simulink model "flightController"  (R2021a)
settings: Solver=ode3  StartTime=0  StopTime=10  FixedStep=Ts  RelTol=1e-3  EnableMultiTasking=on
undefined symbols (not defined in the file): Controller, ControlvsRed, D_ROLL, delays, DiscIntNeverNeededParam, g, I_ROLL, norm_act, Normalization, P_Pitch, P_ROLL, P_Roll, P_Yaw, P_z, PR_Start, save_time, sts_cnames, time_DisYaw, time_stepsX, time_stepsY, time_stepsZ, Ts, Vehicle, x0, x0_f
libraries: deeplib x5
(part 1 of 4)
settings Model: Creator=The MathWorks, Inc.  LastModifiedBy=Eduardo
settings SolverCC: AlgebraicLoopSolver=TrustRegion  MinimalZcImpactIntegration=on
settings DataIOCC: LimitDataPoints=on  SaveFormat=Array  ReturnWorkspaceOutputs=off
settings OptimizationCC: BlockReduction=off  DefaultParameterBehavior=Inlined  BufferReuse=off  PassReuseOutputArgsThreshold=0
settings DebuggingCC: AlgebraicLoopMsg=none  ParameterPrecisionLossMsg=none  ParameterTunabilityLossMsg=error  UnconnectedInputMsg=none  UnconnectedOutputMsg=none  UnconnectedLineMsg=none  BusObjectLabelMismatch=error  SFUnexpectedBacktrackingDiag=warning  SFNoUnconditionalDefaultTransitionDiag=warning  SFExecutionAtInitializationDiag=none  SFMachineParentedDataDiag=warning  ArithmeticOperatorsInVariantConditions=warning
settings HardwareCC: ProdBitPerPointer=32  ProdBitPerSizeT=32  ProdBitPerPtrDiffT=32  ProdLargestAtomicInteger=Long  ProdWordSize=32  ProdHWDeviceType=ARM Compatible->ARM 9
settings ModelReferenceCC: ModelReferenceNumInstancesAllowed=Single  PropagateSignalLabelsOutOfModel=off
settings SFSimCC: SimUseLocalCustomCode=off  CustomCodeUndefinedFunction=UseInterfaceOnly
settings RTWCC: Description=Generic Real-Time Target  GenerateReport=on  RTWUseLocalCustomCode=off  LaunchReport=on
settings CodeAppCC: ForceParamTrailComments=on  MaxIdLength=63  OperatorAnnotations=on  StateflowObjectComments=on  MATLABSourceComments=on
settings GRTTargetCC: TargetLangStandard=C89/C90 (ANSI)
settings ConfigComp: CovMetricSettings=dw  CovSaveCumulativeToWorkspaceVar=on  CovSaveSingleToWorkspaceVar=on  CovExternalEMLEnable=off  CovSFcnEnable=off

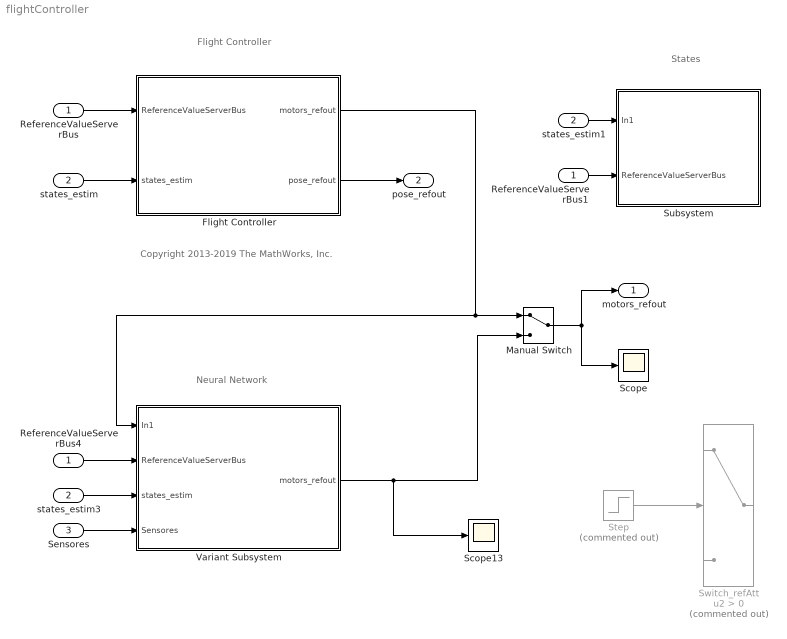
== system flightController ==
  note: States
  note: Copyright 2013-2019 The MathWorks, Inc.
  note: Neural Network
  note: Flight Controller
  ReferenceValueServerBus : Inport  OutDataTypeStr=Bus: CommandBus  BusOutputAsStruct=on
  states_estim : Inport  Port=2  OutDataTypeStr=Bus: statesEstim_t  BusOutputAsStruct=on
  Sensores : Inport  Port=3  OutDataTypeStr=Bus: sensordata_t
  Flight Controller : Subsystem
  Manual Switch : ManualSwitch
  ReferenceValueServerBus1 : InportShadow  OutDataTypeStr=Bus: CommandBus  BusOutputAsStruct=on
  ReferenceValueServerBus4 : InportShadow  OutDataTypeStr=Bus: CommandBus  BusOutputAsStruct=on
  Scope : Scope
  Scope13 : Scope
  Step : Step  Commented=on  Time=0  After=ControlvsRed
  Subsystem : Subsystem
  Switch_refAtt : Switch  Commented=on  Criteria=u2 > Threshold
  Variant Subsystem : Subsystem  Variant=on
  states_estim1 : InportShadow  Port=2  OutDataTypeStr=Bus: statesEstim_t  BusOutputAsStruct=on
  states_estim3 : InportShadow  Port=2  OutDataTypeStr=Bus: statesEstim_t  BusOutputAsStruct=on
  motors_refout : Outport  VectorParamsAs1DForOutWhenUnconnected=off
  pose_refout : Outport  Port=2  VectorParamsAs1DForOutWhenUnconnected=off
  wires:
  ReferenceValueServerBus/1 -> Flight Controller/1(ReferenceValueServerBus)
  states_estim/1 -> Flight Controller/2(states_estim)
  Flight Controller/2(pose_refout) -> pose_refout/1
  Manual Switch/1 -> motors_refout/1, Scope/1
  Flight Controller/1(motors_refout) -> Variant Subsystem/1(In1), Manual Switch/1
  Step/1 -> Switch_refAtt/2
  Variant Subsystem/1(motors_refout) -> Manual Switch/2, Scope13/1
  ReferenceValueServerBus4/1 -> Variant Subsystem/2(ReferenceValueServerBus)
  states_estim3/1 -> Variant Subsystem/3(states_estim)
  Sensores/1 -> Variant Subsystem/4(Sensores)
  ReferenceValueServerBus1/1 -> Subsystem/2(ReferenceValueServerBus)
  states_estim1/1 -> Subsystem/1(In1)

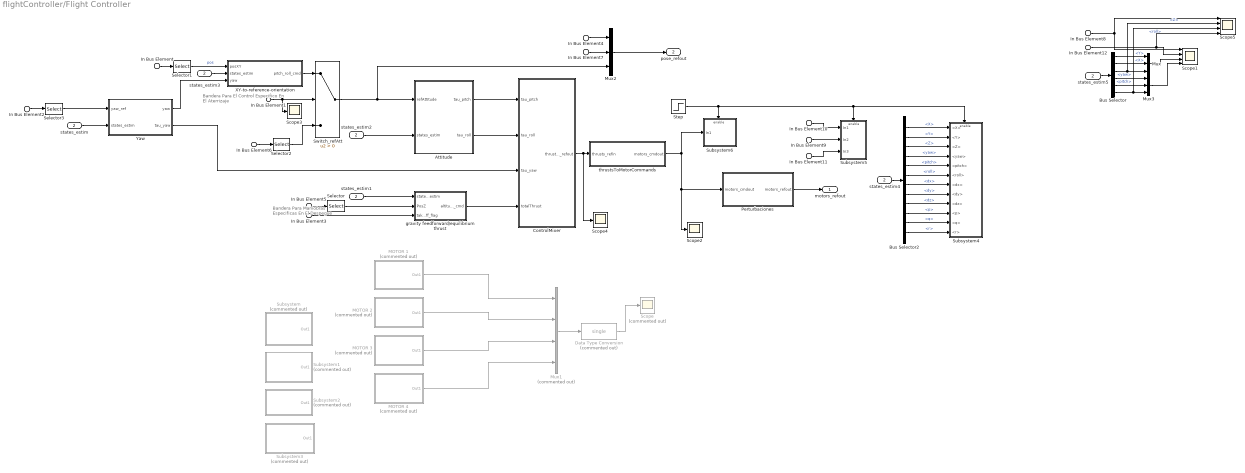
== system flightController/Flight Controller ==
  note: Bandera Para El Control
      | Especifico En El Aterrizaje
  note: Bandera Para
      | Maniobras
      | Especificas
      | En El Despegue
  In Bus Element1 : Inport  PortName=ReferenceValueServerBus  Element=controlModePosVSOrient
  In Bus Element11 : Inport  PortName=ReferenceValueServerBus  Element=controlModePosVSOrient
  In Bus Element{,4..5,8..9} (5 alike) : Inport  PortName=ReferenceValueServerBus  Element=pos_ref
  In Bus Element{2,6..7,10,12} (5 alike) : Inport  PortName=ReferenceValueServerBus  Element=orient_ref
  In Bus Element3 : Inport  PortName=ReferenceValueServerBus  Element=takeoff_flag
  states_estim : Inport  Port=2
  Attitude : Subsystem
  Bus Selector : BusSelector  OutputSignals=Y,X,Z,yaw,pitch,roll
  Bus Selector2 : BusSelector  OutputSignals=X,Y,Z,yaw,pitch,roll,dx,dy,dz,p,q,r
  ControlMixer : Subsystem
  Data Type Conversion : DataTypeConversion  Commented=on  OutDataTypeStr=single
  "MOTOR 1 " : Subsystem  Commented=on  Variant=on  VariantControlMode=label  LabelModeActiveChoice=Choice
  MOTOR 2 : Subsystem  Commented=on  Variant=on  VariantControlMode=label  LabelModeActiveChoice=Choice
  "MOTOR 3 " : Subsystem  Commented=on  Variant=on  VariantControlMode=label  LabelModeActiveChoice=Choice
  "MOTOR 4 " : Subsystem  Commented=on  Variant=on  VariantControlMode=label  LabelModeActiveChoice=Choice
  Mux : Mux  Inputs=3
  Mux1 : Mux  Commented=on
  Mux2 : Mux  Inputs=3
  Mux3 : Mux  Inputs=3
  Perturbaciones : Subsystem
  Scope : Scope  Commented=on
  Scope1 : Scope  NumInputPorts=4
  Scope2 : Scope
  Scope3 : Scope
  Scope4 : Scope
  Scope5 : Scope  NumInputPorts=4
  Selector : Selector  InputPortWidth=3  IndexOptions=Index vector (dialog)  Indices=3  OutputSizes=1
  Selector1 : Selector  InputPortWidth=3  IndexOptions=Index vector (dialog)  Indices=[1 2]  OutputSizes=1
  Selector2 : Selector  InputPortWidth=3  IndexOptions=Index vector (dialog)  Indices=[2 3]  OutputSizes=1
  Selector3 : Selector  InputPortWidth=3  IndexOptions=Index vector (dialog)  Indices=1  OutputSizes=1
  Step : Step  Time=save_time
  Subsystem : Subsystem  Commented=on
  Subsystem1 : Subsystem  Commented=on
  Subsystem2 : Subsystem  Commented=on
  Subsystem3 : Subsystem  Commented=on
  Subsystem4 : Subsystem
  Subsystem5 : Subsystem
  Subsystem6 : Subsystem
  Switch_refAtt : Switch  Criteria=u2 > Threshold
  XY-to-reference-orientation : Subsystem
  Yaw : Subsystem
  gravity feedforward/equilibrium thrust : Subsystem
  states_estim{1..5} (5 alike) : InportShadow  Port=2
  thrustsToMotorCommands : Subsystem
  motors_refout : Outport  VectorParamsAs1DForOutWhenUnconnected=off
  pose_refout : Outport  Port=2  VectorParamsAs1DForOutWhenUnconnected=off
  wires:
  In Bus Element1/1 -> Scope3/1, Switch_refAtt/2
  XY-to-reference-orientation/1(pitch_roll_cmd) -> Switch_refAtt/1
  In Bus Element2/1 -> Selector3/1
  In Bus Element/1 -> Selector1/1
  Selector3/1 -> Yaw/1(yaw_ref)
  Selector1/1 -> XY-to-reference-orientation/1(posXY)  "pos"
  ControlMixer/1(thrusts_refout) -> thrustsToMotorCommands/1(thrusts_refin), Scope4/1
  states_estim/1 -> Yaw/2(states_estim)
  Switch_refAtt/1 -> Attitude/1(refAttitude), Mux2/3
  Yaw/1(yaw) -> XY-to-reference-orientation/3(yaw)
  gravity feedforward/equilibrium thrust/1(altitude_cmd) -> ControlMixer/4(totalThrust)
  Attitude/1(tau_pitch) -> ControlMixer/1(tau_pitch)
  Attitude/2(tau_roll) -> ControlMixer/2(tau_roll)
  Yaw/2(tau_yaw) -> ControlMixer/3(tau_yaw)
  states_estim1/1 -> gravity feedforward/equilibrium thrust/1(states_estim)
  states_estim2/1 -> Attitude/2(states_estim)
  states_estim3/1 -> XY-to-reference-orientation/2(states_estim)
  In Bus Element4/1 -> Mux2/1
  Selector/1 -> gravity feedforward/equilibrium thrust/2(PosZ)
  In Bus Element5/1 -> Selector/1
  In Bus Element6/1 -> Selector2/1
  Selector2/1 -> Switch_refAtt/3
  In Bus Element7/1 -> Mux2/2
  Mux1/1 -> Data Type Conversion/1
  "MOTOR 1 "/1(Out1) -> Mux1/1
  MOTOR 2/1(Out1) -> Mux1/2
  "MOTOR 3 "/1(Out1) -> Mux1/3
  "MOTOR 4 "/1(Out1) -> Mux1/4
  Mux2/1 -> pose_refout/1
  Data Type Conversion/1 -> Scope/1
  states_estim4/1 -> Bus Selector2/1
  In Bus Element8/1 -> Scope5/1, Scope1/1
  states_estim5/1 -> Bus Selector/1
  Bus Selector/1 -> Mux/1  "<Y>"
  Bus Selector/3 -> Scope5/2, Mux/3  "<Z>"
  Bus Selector/4 -> Mux3/1  "<yaw>"
  Bus Selector/5 -> Mux3/2  "<pitch>"
  Bus Selector/6 -> Scope5/3, Mux3/3  "<roll>"
  In Bus Element3/1 -> gravity feedforward/equilibrium thrust/3(takeoff_flag)
  Bus Selector2/1 -> Subsystem4/1(<X>)  "<X>"
  Bus Selector2/2 -> Subsystem4/2(<Y>)  "<Y>"
  Bus Selector2/3 -> Subsystem4/3(<Z>)  "<Z>"
  Bus Selector2/4 -> Subsystem4/4(<yaw>)  "<yaw>"
  Bus Selector2/5 -> Subsystem4/5(<pitch>)  "<pitch>"
  Bus Selector2/6 -> Subsystem4/6(<roll>)  "<roll>"
  Bus Selector2/7 -> Subsystem4/7(<dx>)  "<dx>"
  Bus Selector2/8 -> Subsystem4/8(<dy>)  "<dy>"
  Bus Selector2/9 -> Subsystem4/9(<dz>)  "<dz>"
  Bus Selector2/10 -> Subsystem4/10(<p>)  "<p>"
  Bus Selector2/11 -> Subsystem4/11(<q>)  "<q>"
  Bus Selector2/12 -> Subsystem4/12(<r>)  "<r>"
  Step/1 -> Subsystem6/Enable, Subsystem5/Enable, Subsystem4/Enable
  In Bus Element10/1 -> Subsystem5/1(In1)
  In Bus Element9/1 -> Subsystem5/2(In2)
  In Bus Element11/1 -> Subsystem5/3(In3)
  In Bus Element12/1 -> Scope5/4, Scope1/2
  thrustsToMotorCommands/1(motors_cmdout) -> Perturbaciones/1(motors_cmdout), Scope2/1, Subsystem6/1(In1)
  Bus Selector/2 -> Mux/2  "<X>"
  Mux/1 -> Scope1/3
  Mux3/1 -> Scope1/4
  Perturbaciones/1(motors_refout) -> motors_refout/1

== system flightController/Subsystem ==
  note: Yaw
  note: X
  note: Y
  note: Z
  note: Pitch
  note: Roll
  In1 : Inport
  In Bus Element2 : Inport  Port=2  PortName=ReferenceValueServerBus  Element=orient_ref
  In Bus Element5 : Inport  Port=2  PortName=ReferenceValueServerBus  Element=orient_ref
  In Bus Element6 : Inport  Port=2  PortName=ReferenceValueServerBus  Element=orient_ref
  In Bus Element1 : Inport  Port=2  PortName=ReferenceValueServerBus  Element=pos_ref
  In Bus Element3 : Inport  Port=2  PortName=ReferenceValueServerBus  Element=pos_ref
  In Bus Element4 : Inport  Port=2  PortName=ReferenceValueServerBus  Element=pos_ref
  Bus Selector2 : BusSelector  OutputSignals=X,Y,Z,yaw,pitch,roll
  Mux{,1..5} (6 alike) : Mux  Inputs=2
  Scope1 : Scope  NumInputPorts=6
  Selector1 : Selector  InputPortWidth=3  IndexOptions=Index vector (dialog)  Indices=1  OutputSizes=1
  Selector2 : Selector  InputPortWidth=3  IndexOptions=Index vector (dialog)  Indices=2  OutputSizes=1
  Selector3 : Selector  InputPortWidth=3  IndexOptions=Index vector (dialog)  Indices=1  OutputSizes=1
  Selector4 : Selector  InputPortWidth=3  IndexOptions=Index vector (dialog)  Indices=3  OutputSizes=1
  Selector5 : Selector  InputPortWidth=3  IndexOptions=Index vector (dialog)  Indices=2  OutputSizes=1
  Selector6 : Selector  InputPortWidth=3  IndexOptions=Index vector (dialog)  Indices=3  OutputSizes=1
  wires:
  In Bus Element2/1 -> Selector3/1
  In1/1 -> Bus Selector2/1
  Bus Selector2/1 -> Mux/1  "<X>"
  Bus Selector2/2 -> Mux1/1  "<Y>"
  Bus Selector2/3 -> Mux2/1  "<Z>"
  Bus Selector2/4 -> Mux3/1  "<yaw>"
  Bus Selector2/5 -> Mux4/1  "<pitch>"
  Bus Selector2/6 -> Mux5/1  "<roll>"
  In Bus Element1/1 -> Selector1/1
  In Bus Element3/1 -> Selector2/1
  In Bus Element4/1 -> Selector4/1
  In Bus Element5/1 -> Selector5/1
  In Bus Element6/1 -> Selector6/1
  Selector1/1 -> Mux/2  "X_ref"
  Selector2/1 -> Mux1/2  "Y_ref"
  Selector4/1 -> Mux2/2  "Z_ref"
  Selector3/1 -> Mux3/2  "Yaw_ref"
  Selector5/1 -> Mux4/2  "Pitch_ref"
  Selector6/1 -> Mux5/2  "Roll_ref"
  Mux/1 -> Scope1/1
  Mux2/1 -> Scope1/3
  Mux5/1 -> Scope1/6
  Mux4/1 -> Scope1/5
  Mux3/1 -> Scope1/4
  Mux1/1 -> Scope1/2

== system flightController/Variant Subsystem ==
  note: 1) Add Subsystem or Model blocks as valid variant choices.
      | 2) You cannot connect blocks at this level. At simulation, connectivity is automatically
      | determined, based on the active variant and port name matching.
  In1 : Inport
  ReferenceValueServerBus : Inport  Port=2
  states_estim : Inport  Port=3
  Sensores : Inport  Port=4
  ANN : Subsystem  VariantControl=ANN
  ANN_Feedback : Subsystem  VariantControl=ANN_Feedback
  LSTM : Subsystem  VariantControl=LSTM
  motors_refout : Outport

== system flightController/Flight Controller/Attitude ==
  note: [0.002;0.01119]
  note: 0.001616
  note: OC [P]
  note: OPSO [P]
  note: [0.013;0.06656]
  note: 0.005
  note: [0.013;0.01]
  note: [0.002; 0.0028]
  note: 0.001
  note: OC [I]
  note: ATTITUDE
  note: 0.01
  note: OPSO [I]
  note: OC [D]
  note: OPSO [D]
  refAttitude : Inport
  states_estim : Inport  Port=2
  Add : Sum  Inputs=+-
  Bus Selector3 : BusSelector  OutputSignals=pitch,roll
  Bus Selector4 : BusSelector  OutputSignals=q,p
  D_pr : Gain  Gain=[0.002; D_ROLL]
  Delay : Delay  DelayLength=1  InitialCondition=0
  Demux : Demux  Outputs=2
  Discrete-Time Integrator : DiscreteIntegrator  SampleTime=Ts  LimitOutput=on  UpperSaturationLimit=2  LowerSaturationLimit=-2  ICPrevOutput=DiscIntNeverNeededParam  ICPrevScaledInput=DiscIntNeverNeededParam
  I_pr : Gain  Gain=I_ROLL
  Mux : Mux  Inputs=2
  Mux1 : Mux  Inputs=2
  P_pr : Gain  Gain=[0.013;P_ROLL]
  Scope : Scope
  Scope{1..5} (5 alike) : Scope  NumInputPorts=2
  Sum16 : Sum  Inputs=++-  AccumDataTypeStr=single  OutDataTypeStr=single  SaturateOnIntegerOverflow=on
  Sum19 : Sum  Inputs=+-|
  antiWU_Gain : Gain  Gain=0.001
  tau_pitch : Outport  VectorParamsAs1DForOutWhenUnconnected=off
  tau_roll : Outport  Port=2  VectorParamsAs1DForOutWhenUnconnected=off
  wires:
  Sum16/1 -> Demux/1  "P_pr"
  antiWU_Gain/1 -> Add/2
  Add/1 -> Discrete-Time Integrator/1
  Bus Selector3/1 -> Mux/1  "<pitch>"
  Bus Selector4/1 -> Mux1/1  "<q>"
  P_pr/1 -> Scope3/2, Sum16/1
  I_pr/1 -> Sum16/2, Scope/1
  Sum19/1 -> Add/1, Scope2/2, P_pr/1  "pitch/roll error"
  Discrete-Time Integrator/1 -> Delay/1, I_pr/1
  Delay/1 -> antiWU_Gain/1
  Demux/1 -> tau_pitch/1  "tau_pitch"
  Demux/2 -> tau_roll/1
  D_pr/1 -> Scope5/1, Sum16/3
  states_estim/1 -> Bus Selector3/1, Bus Selector4/1
  refAttitude/1 -> Sum19/1
  Mux/1 -> Sum19/2
  Bus Selector3/2 -> Scope1/1, Mux/2  "<roll>"
  Mux1/1 -> Scope4/1, D_pr/1
  Bus Selector4/2 -> Scope1/2, Mux1/2  "<p>"

== system flightController/Flight Controller/ControlMixer ==
  tau_pitch : Inport
  tau_roll : Inport  Port=2
  tau_yaw : Inport  Port=3
  totalThrust : Inport  Port=4
  Mux2 : Mux
  Product : Product  Multiplication=Matrix(*)  RndMeth=Zero
  TorqueTotalThrustToThrustPerMotor : Constant  Value=Controller.Q2Ts  OutDataTypeStr=single
  thrusts_refout : Outport  VectorParamsAs1DForOutWhenUnconnected=off
  wires:
  Product/1 -> thrusts_refout/1
  tau_roll/1 -> Mux2/4
  tau_pitch/1 -> Mux2/3
  tau_yaw/1 -> Mux2/2
  totalThrust/1 -> Mux2/1
  TorqueTotalThrustToThrustPerMotor/1 -> Product/1
  Mux2/1 -> Product/2

== system flightController/Flight Controller/MOTOR 1  ==
  note: 1) Add Subsystem or Model blocks as valid variant choices.
      | 2) You cannot connect blocks at this level. At simulation, connectivity is automatically
      | determined, based on the active variant and port name matching.
  "PITCH " : Subsystem  VariantControl=Choice_3
  "ROLL " : Subsystem  VariantControl=Choice
  SUBIR : Subsystem  VariantControl=Choice_1
  YAW : Subsystem  VariantControl=Choice_2
  Out1 : Outport

== system flightController/Flight Controller/MOTOR 2 ==
  note: 1) Add Subsystem or Model blocks as valid variant choices.
      | 2) You cannot connect blocks at this level. At simulation, connectivity is automatically
      | determined, based on the active variant and port name matching.
  "PITCH " : Subsystem  VariantControl=Choice_3
  ROLL : Subsystem  VariantControl=Choice
  SUBIR : Subsystem  VariantControl=Choice_1
  YAW : Subsystem  VariantControl=Choice_2
  Out1 : Outport

== system flightController/Flight Controller/MOTOR 3  ==
  note: 1) Add Subsystem or Model blocks as valid variant choices.
      | 2) You cannot connect blocks at this level. At simulation, connectivity is automatically
      | determined, based on the active variant and port name matching.
  "PITCH " : Subsystem  VariantControl=Choice_3
  "ROLL " : Subsystem  VariantControl=Choice
  SUBIR : Subsystem  VariantControl=Choice_1
  YAW : Subsystem  VariantControl=Choice_2
  Out1 : Outport

== system flightController/Flight Controller/MOTOR 4  ==
  note: 1) Add Subsystem or Model blocks as valid variant choices.
      | 2) You cannot connect blocks at this level. At simulation, connectivity is automatically
      | determined, based on the active variant and port name matching.
  "PITCH " : Subsystem  VariantControl=Choice_3
  "ROLL " : Subsystem  VariantControl=Choice
  SUBIR : Subsystem  VariantControl=Choice_1
  YAW : Subsystem  VariantControl=Choice_2
  Out1 : Outport

== system flightController/Flight Controller/Perturbaciones ==
  motors_cmdout : Inport
  Data Type Conversion : DataTypeConversion  OutDataTypeStr=single
  Demux : Demux
  Mux1 : Mux
  Perturbaciones en Pitch : Subsystem
  Perturbaciones en Roll : Subsystem
  Perturbaciones en Yaw : Subsystem
  Perturbaciones en Z : Subsystem
  Scope6 : Scope  NumInputPorts=4
  Sum : Sum  Inputs=|++++
  Sum1 : Sum  Inputs=|++-+
  Sum2 : Sum  Inputs=|++
  Sum3 : Sum  Inputs=|++-+
  motors_refout : Outport
  wires:
  Perturbaciones en Z/1(Out1) -> Sum1/3, Sum/4, Sum2/2, Sum3/3
  Mux1/1 -> Data Type Conversion/1
  Demux/4 -> Sum3/1
  Demux/1 -> Sum/1
  Perturbaciones en Roll/1(Out1) -> Sum/3, Sum1/2, Scope6/4
  Sum2/1 -> Mux1/3
  Sum3/1 -> Mux1/4
  Perturbaciones en Pitch/1(Out1) -> Scope6/2, Sum3/2, Sum/2, Scope6/1
  Sum1/1 -> Mux1/2
  Demux/2 -> Sum1/1
  Demux/3 -> Sum2/1
  Sum/1 -> Mux1/1
  motors_cmdout/1 -> Demux/1
  Data Type Conversion/1 -> motors_refout/1
  Perturbaciones en Yaw/1(Out1) -> Scope6/3, Sum3/4, Sum1/4

== system flightController/Flight Controller/Subsystem ==
  note: SI
  Pulse Generator : DiscretePulseGenerator  Commented=on  PulseType=Time based  Amplitude=50  Period=1.5  PulseWidth=50
  Pulse Generator1 : DiscretePulseGenerator  Commented=on  PulseType=Time based  Amplitude=30  Period=1.5  PulseWidth=50
  Step : Step  Commented=on  Time=0.001  Before=30  After=350
  Step1 : Step  Commented=on  Time=0.001  Before=30  After=350
  Step10 : Step  Commented=on  Time=0.001  Before=30  After=380
  Step11 : Step  Commented=on  Time=1.5  Before=1  After=0
  Step2 : Step  Commented=on  Time=0.001  Before=30  After=420
  Step3 : Step  Commented=on  Time=1.5  Before=1  After=0
  Step4 : Step  Commented=on  Time=0.001  Before=-30  After=237
  Step5 : Step  Commented=on  Time=3  Before=1  After=0
  Step6 : Step  Time=0.001  Before=30  After=350
  Step7 : Step  Time=0.001  Before=30  After=380
  Step8 : Step  Time=1.5  Before=1  After=0
  Step9 : Step  Commented=on  Time=0.001  Before=30  After=350
  Sum : Sum  Commented=on  Inputs=|+-
  Sum1 : Sum  Commented=on  Inputs=|+-
  Switch : Switch  Commented=on  Criteria=u2 > Threshold
  Switch1 : Switch  Commented=on  Criteria=u2 > Threshold
  Switch2 : Switch  Criteria=u2 > Threshold
  Switch3 : Switch  Commented=on  Criteria=u2 > Threshold
  Out1 : Outport
  wires:
  Step/1 -> Switch/1
  Step5/1 -> Switch/2
  Pulse Generator/1 -> Sum/2
  Step2/1 -> Sum/1
  Sum/1 -> Switch/3
  Step1/1 -> Switch1/1
  Step3/1 -> Switch1/2
  Step4/1 -> Sum1/1
  Sum1/1 -> Switch1/3
  Pulse Generator1/1 -> Sum1/2
  Step6/1 -> Switch2/1
  Step8/1 -> Switch2/2
  Step7/1 -> Switch2/3
  Step11/1 -> Switch3/2
  Step10/1 -> Switch3/3
  Step9/1 -> Switch3/1
  Switch2/1 -> Out1/1

== system flightController/Flight Controller/Subsystem1 ==
  note: SI
  Pulse Generator : DiscretePulseGenerator  Commented=on  PulseType=Time based  Amplitude=50  Period=1.5  PulseWidth=50
  Pulse Generator1 : DiscretePulseGenerator  Commented=on  PulseType=Time based  Amplitude=30  Period=1.5  PulseWidth=50
  Step1 : Step  Commented=on  Time=0.001  Before=-30  After=-280
  Step10 : Step  Commented=on  Time=0.001  Before=-30  After=-310
  Step{2,4,8,11} (4 alike) : Step  Commented=on  Time=0.001  Before=-30  After=-350
  Step12 : Step  Commented=on  Time=1.5
  Step3 : Step  Commented=on  Time=3
  Step5 : Step  Commented=on  Time=1.5
  Step6 : Step  Commented=on  Time=0.001  Before=-30  After=-380
  Step7 : Step  Commented=on  Time=0.001  Before=-30  After=-237
  Step9 : Step  Commented=on  Time=1.5
  Sum : Sum  Commented=on  Inputs=|++
  Sum1 : Sum  Commented=on  Inputs=|++
  Switch{,1..3} (4 alike) : Switch  Commented=on  Criteria=u2 > Threshold
  Out1 : Outport
  wires:
  Step5/1 -> Switch/2
  Step4/1 -> Switch/3
  Sum1/1 -> Switch/1
  Step3/1 -> Switch1/2
  Step2/1 -> Switch1/3
  Pulse Generator/1 -> Sum/1
  Step1/1 -> Sum/2
  Sum/1 -> Switch1/1
  Pulse Generator1/1 -> Sum1/2
  Step7/1 -> Sum1/1
  Step8/1 -> Switch2/3
  Step6/1 -> Switch2/1
  Step9/1 -> Switch2/2
  Step12/1 -> Switch3/2
  Step11/1 -> Switch3/3
  Step10/1 -> Switch3/1
  Switch1/1 -> Out1/1

== system flightController/Flight Controller/Subsystem2 ==
  note: SI
  Pulse Generator : DiscretePulseGenerator  PulseType=Time based  Amplitude=50  Period=1.5  PulseWidth=50
  Pulse Generator1 : DiscretePulseGenerator  Commented=on  PulseType=Time based  Amplitude=30  Period=1.5  PulseWidth=50
  Step : Step  Commented=on  Time=0.001  Before=30  After=350
  Step1 : Step  Time=0.001  Before=30  After=350
  Step10 : Step  Commented=on  Time=0.001  Before=30  After=310
  Step11 : Step  Commented=on  Time=1.5  Before=1  After=0
  Step2 : Step  Time=0.001  Before=30  After=420
  Step3 : Step  Time=3  Before=1  After=0
  Step4 : Step  Commented=on  Time=0.001  Before=-30  After=237
  Step5 : Step  Commented=on  Time=1.5  Before=1  After=0
  Step6 : Step  Commented=on  Time=0.001  Before=30  After=350
  Step7 : Step  Commented=on  Time=0.001  Before=30  After=310
  Step8 : Step  Commented=on  Time=1.5  Before=1  After=0
  Step9 : Step  Commented=on  Time=0.001  Before=30  After=350
  Sum : Sum  Inputs=|+-
  Sum1 : Sum  Commented=on  Inputs=|+-
  Switch : Switch  Commented=on  Criteria=u2 > Threshold
  Switch1 : Switch  Criteria=u2 > Threshold
  Switch2 : Switch  Commented=on  Criteria=u2 > Threshold
  Switch3 : Switch  Commented=on  Criteria=u2 > Threshold
  Out1 : Outport
  wires:
  Step5/1 -> Switch/2
  Step/1 -> Switch/1
  Step1/1 -> Switch1/1
  Step3/1 -> Switch1/2
  Step2/1 -> Sum/1
  Sum/1 -> Switch1/3
  Pulse Generator/1 -> Sum/2
  Pulse Generator1/1 -> Sum1/2
  Step4/1 -> Sum1/1
  Sum1/1 -> Switch/3
  Step8/1 -> Switch2/2
  Step6/1 -> Switch2/1
  Step7/1 -> Switch2/3
  Step9/1 -> Switch3/1
  Step11/1 -> Switch3/2
  Step10/1 -> Switch3/3
  Switch1/1 -> Out1/1

== system flightController/Flight Controller/Subsystem3 ==
  note: SI
  Pulse Generator : DiscretePulseGenerator  PulseType=Time based  Amplitude=50  Period=1.5  PulseWidth=50
  Pulse Generator1 : DiscretePulseGenerator  Commented=on  PulseType=Time based  Amplitude=30  Period=1.5  PulseWidth=50
  Step1 : Step  Time=0.001  Before=-30  After=-280
  Step10 : Step  Commented=on  Time=0.001  Before=-30  After=-380
  Step11 : Step  Commented=on  Time=0.001  Before=-30  After=-350
  Step12 : Step  Commented=on  Time=1.5
  Step2 : Step  Time=0.001  Before=-30  After=-350
  Step3 : Step  Time=3
  Step4 : Step  Commented=on  Time=0.001  Before=-30  After=-350
  Step5 : Step  Commented=on  Time=1.5
  Step6 : Step  Commented=on  Time=0.001  Before=-30  After=-310
  Step7 : Step  Commented=on  Time=0.001  Before=-30  After=-237
  Step8 : Step  Commented=on  Time=0.001  Before=-30  After=-350
  Step9 : Step  Commented=on  Time=1.5
  Sum : Sum  Inputs=|++
  Sum1 : Sum  Commented=on  Inputs=|++
  Switch : Switch  Commented=on  Criteria=u2 > Threshold
  Switch1 : Switch  Criteria=u2 > Threshold
  Switch2 : Switch  Commented=on  Criteria=u2 > Threshold
  Switch3 : Switch  Commented=on  Criteria=u2 > Threshold
  Out1 : Outport
  wires:
  Step5/1 -> Switch/2
  Step4/1 -> Switch/3
  Step3/1 -> Switch1/2
  Step2/1 -> Switch1/3
  Step1/1 -> Sum/2
  Pulse Generator/1 -> Sum/1
  Sum/1 -> Switch1/1
  Step7/1 -> Sum1/1
  Pulse Generator1/1 -> Sum1/2
  Sum1/1 -> Switch/1
  Step6/1 -> Switch2/1
  Step8/1 -> Switch2/3
  Step9/1 -> Switch2/2
  Step12/1 -> Switch3/2
  Step11/1 -> Switch3/3
  Step10/1 -> Switch3/1
  Switch1/1 -> Out1/1

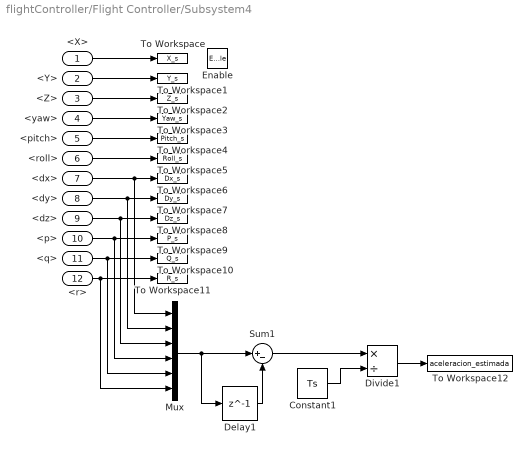
== system flightController/Flight Controller/Subsystem4 ==
  <X> : Inport
  <Y> : Inport  Port=2
  <Z> : Inport  Port=3
  <yaw> : Inport  Port=4
  <pitch> : Inport  Port=5
  <roll> : Inport  Port=6
  <dx> : Inport  Port=7
  <dy> : Inport  Port=8
  <dz> : Inport  Port=9
  <p> : Inport  Port=10
  <q> : Inport  Port=11
  <r> : Inport  Port=12
  Enable : EnablePort
  Constant1 : Constant  Value=Ts
  Delay1 : Delay  DelayLength=1  InitialCondition=0
  Divide1 : Product  Inputs=*/
  Mux : Mux  Inputs=6
  Sum1 : Sum  Inputs=|+-
  To Workspace : ToWorkspace  VariableName=X_s  SaveFormat=Structure With Time  SampleTime=-1
      settings: Save2DSignal=2-D array (concatenate along first dimension)
  To Workspace1 : ToWorkspace  VariableName=Y_s  SaveFormat=Structure  SampleTime=-1
      settings: Save2DSignal=2-D array (concatenate along first dimension)
  To Workspace10 : ToWorkspace  VariableName=Q_s  SaveFormat=Structure  SampleTime=-1
      settings: Save2DSignal=2-D array (concatenate along first dimension)
  To Workspace11 : ToWorkspace  VariableName=R_s  SaveFormat=Structure  SampleTime=-1
      settings: Save2DSignal=2-D array (concatenate along first dimension)
  To Workspace12 : ToWorkspace  VariableName=aceleracion_estimada  SaveFormat=Structure  SampleTime=-1
      settings: Save2DSignal=2-D array (concatenate along first dimension)
  To Workspace2 : ToWorkspace  VariableName=Z_s  SaveFormat=Structure  SampleTime=-1
      settings: Save2DSignal=2-D array (concatenate along first dimension)
  To Workspace3 : ToWorkspace  VariableName=Yaw_s  SaveFormat=Structure  SampleTime=-1
      settings: Save2DSignal=2-D array (concatenate along first dimension)
  To Workspace4 : ToWorkspace  VariableName=Pitch_s  SaveFormat=Structure With Time  SampleTime=-1
      settings: Save2DSignal=2-D array (concatenate along first dimension)
  To Workspace5 : ToWorkspace  VariableName=Roll_s  SaveFormat=Structure  SampleTime=-1
      settings: Save2DSignal=2-D array (concatenate along first dimension)
  To Workspace6 : ToWorkspace  VariableName=Dx_s  SaveFormat=Structure  SampleTime=-1
      settings: Save2DSignal=2-D array (concatenate along first dimension)
  To Workspace7 : ToWorkspace  VariableName=Dy_s  SaveFormat=Structure  SampleTime=-1
      settings: Save2DSignal=2-D array (concatenate along first dimension)
  To Workspace8 : ToWorkspace  VariableName=Dz_s  SaveFormat=Structure  SampleTime=-1
      settings: Save2DSignal=2-D array (concatenate along first dimension)
  To Workspace9 : ToWorkspace  VariableName=P_s  SaveFormat=Structure  SampleTime=-1
      settings: Save2DSignal=2-D array (concatenate along first dimension)
  wires:
  <Z>/1 -> To Workspace2/1
  <roll>/1 -> To Workspace5/1
  <dz>/1 -> Mux/3, To Workspace8/1
  <Y>/1 -> To Workspace1/1
  <yaw>/1 -> To Workspace3/1
  <pitch>/1 -> To Workspace4/1
  <p>/1 -> Mux/4, To Workspace9/1
  <dx>/1 -> Mux/1, To Workspace6/1
  <q>/1 -> Mux/5, To Workspace10/1
  <r>/1 -> To Workspace11/1, Mux/6
  <dy>/1 -> Mux/2, To Workspace7/1
  <X>/1 -> To Workspace/1
  Sum1/1 -> Divide1/1
  Constant1/1 -> Divide1/2
  Delay1/1 -> Sum1/2
  Divide1/1 -> To Workspace12/1
  Mux/1 -> Sum1/1, Delay1/1

== system flightController/Flight Controller/Subsystem5 ==
  In1 : Inport
  In2 : Inport  Port=2
  In3 : Inport  Port=3
  Enable : EnablePort
  Constant : Constant  Value=Ts
  Constant1 : Constant  Value=Ts
  Delay1 : Delay  DelayLength=1  InitialCondition=0
  Delay2 : Delay  DelayLength=1  InitialCondition=0
  Divide : Product  Inputs=*/
  Divide1 : Product  Inputs=*/
  Scope : Scope  NumInputPorts=2
  Sum : Sum  Inputs=|+-
  Sum1 : Sum  Inputs=|+-
  To Workspace1 : ToWorkspace  VariableName=FlgRefOrient  SaveFormat=Structure  SampleTime=-1
      settings: Save2DSignal=2-D array (concatenate along first dimension)
  To Workspace12 : ToWorkspace  VariableName=pos_r  SaveFormat=Structure  SampleTime=-1
      settings: Save2DSignal=2-D array (concatenate along first dimension)
  To Workspace13 : ToWorkspace  VariableName=orient_r  SaveFormat=Structure  SampleTime=-1
      settings: Save2DSignal=2-D array (concatenate along first dimension)
  To Workspace2 : ToWorkspace  VariableName=v_pos_r  SaveFormat=Structure  SampleTime=-1
      settings: Save2DSignal=2-D array (concatenate along first dimension)
  To Workspace3 : ToWorkspace  VariableName=v_orient_r  SaveFormat=Structure  SampleTime=-1
      settings: Save2DSignal=2-D array (concatenate along first dimension)
  wires:
  In3/1 -> To Workspace1/1
  Divide/1 -> Scope/2, To Workspace3/1
  Sum/1 -> Divide/1
  In1/1 -> Delay2/1, Sum/1, To Workspace13/1
  Constant/1 -> Divide/2
  Delay2/1 -> Sum/2
  Delay1/1 -> Sum1/2
  Constant1/1 -> Divide1/2
  In2/1 -> Delay1/1, Sum1/1, To Workspace12/1
  Sum1/1 -> Divide1/1
  Divide1/1 -> Scope/1, To Workspace2/1

== system flightController/Flight Controller/Subsystem6 ==
  In1 : Inport
  Enable : EnablePort
  To Workspace14 : ToWorkspace  VariableName=TM  SaveFormat=Structure  SampleTime=-1
      settings: Save2DSignal=2-D array (concatenate along first dimension)
  wires:
  In1/1 -> To Workspace14/1

== system flightController/Flight Controller/XY-to-reference-orientation ==
  posXY : Inport
  states_estim : Inport  Port=2
  yaw : Inport  Port=3
  Bus Selector1 : BusSelector  OutputSignals=X,Y
  Bus Selector2 : BusSelector  OutputSignals=dx,dy
  D_xy : Gain  Gain=[0.1, -0.1]  ParamDataTypeStr=single  OutDataTypeStr=single  SaturateOnIntegerOverflow=on
  Gain : Gain  Gain=-1
  Matrix Concatenate : Concatenate  Mode=Multidimensional array  ConcatenateDimension=2
  Mux : Mux  Inputs=2
  Mux1 : Mux  Inputs=2
  P_xy : Gain  Gain=[-0.24,0.24]  ParamDataTypeStr=single  OutDataTypeStr=single  SaturateOnIntegerOverflow=on
  Product : Product  Multiplication=Matrix(*)  OutDataTypeStr=single  RndMeth=Zero
  Saturation : Saturate  UpperLimit=3  LowerLimit=-3  OutDataTypeStr=single
  Sum17 : Sum  Inputs=+-|  AccumDataTypeStr=single
  Sum18 : Sum  Inputs=|++  AccumDataTypeStr=single  OutDataTypeStr=single  SaturateOnIntegerOverflow=on
  Trigonometric Function : Trigonometry  Operator=sincos
  Vector Concatenate : Concatenate
  Vector Concatenate1 : Concatenate
  pitch_roll_cmd : Outport  VectorParamsAs1DForOutWhenUnconnected=off
  wires:
  yaw/1 -> Trigonometric Function/1
  Saturation/1 -> P_xy/1
  P_xy/1 -> Sum18/1
  Sum17/1 -> Product/2  "XY error"
  posXY/1 -> Sum17/1
  Bus Selector2/1 -> Mux1/1  "<dx>"
  states_estim/1 -> Bus Selector1/1, Bus Selector2/1
  Sum18/1 -> pitch_roll_cmd/1  "pitch/roll cmd"
  D_xy/1 -> Sum18/2
  Bus Selector1/1 -> Mux/1  "<X>"
  Product/1 -> Saturation/1
  Trigonometric Function/1 -> Gain/1, Vector Concatenate1/1
  Trigonometric Function/2 -> Vector Concatenate1/2, Vector Concatenate/1
  Gain/1 -> Vector Concatenate/2
  Vector Concatenate/1 -> Matrix Concatenate/1
  Vector Concatenate1/1 -> Matrix Concatenate/2
  Matrix Concatenate/1 -> Product/1
  Bus Selector1/2 -> Mux/2  "<Y>"
  Mux/1 -> Sum17/2
  Mux1/1 -> D_xy/1
  Bus Selector2/2 -> Mux1/2  "<dy>"

== system flightController/Flight Controller/Yaw ==
  yaw_ref : Inport
  states_estim : Inport  Port=2
  Bus Selector5 : BusSelector  OutputSignals=yaw,r
  D_yaw : Gain  Gain=0.3*0.004
  P_yaw : Gain  Gain=0.004  ParamDataTypeStr=single  OutDataTypeStr=single
  Sum1 : Sum  Inputs=+-|  AccumDataTypeStr=single  OutDataTypeStr=single  SaturateOnIntegerOverflow=on
  Sum2 : Sum  Inputs=|+-
  yaw : Outport  VectorParamsAs1DForOutWhenUnconnected=off
  tau_yaw : Outport  Port=2  VectorParamsAs1DForOutWhenUnconnected=off
  wires:
  D_yaw/1 -> Sum2/2
  P_yaw/1 -> Sum2/1
  Bus Selector5/2 -> D_yaw/1  "<r>"
  Sum1/1 -> P_yaw/1
  states_estim/1 -> Bus Selector5/1
  Sum2/1 -> tau_yaw/1
  Bus Selector5/1 -> yaw/1, Sum1/2  "<yaw>"
  yaw_ref/1 -> Sum1/1

== system flightController/Flight Controller/gravity feedforward//equilibrium thrust ==
  note: ALTITUDE
  states_estim : Inport
  PosZ : Inport  Port=2
  takeoff_flag : Inport  Port=3
  Bus Selector6 : BusSelector  OutputSignals=Z,dz
  D_z : Gain  Gain=0.3  ParamDataTypeStr=single  OutDataTypeStr=single  SaturateOnIntegerOverflow=on
  P_z : Gain  Gain=0.8  ParamDataTypeStr=single  OutDataTypeStr=single  SaturateOnIntegerOverflow=on
  SaturationThrust : Saturate  UpperLimit=4*Controller.totalThrustMaxRelative*Controller.motorsThrustPerMotorMax  LowerLimit=-4*Controller.totalThrustMaxRelative*Controller.motorsThrustPerMotorMax  OutDataTypeStr=single
  Sum15 : Sum  Inputs=|+-  AccumDataTypeStr=single  OutDataTypeStr=single  SaturateOnIntegerOverflow=on
  Sum3 : Sum  Inputs=+-|  AccumDataTypeStr=single  OutDataTypeStr=single  SaturateOnIntegerOverflow=on
  Sum4 : Sum  Inputs=++|  AccumDataTypeStr=single  OutDataTypeStr=single  SaturateOnIntegerOverflow=on
  TakeoffOrControl_Switch : Switch  Criteria=u2 > Threshold
  takeoff_gain : Gain  Gain=Controller.takeoffGain  ParamDataTypeStr=single  OutDataTypeStr=single  SaturateOnIntegerOverflow=on
  w0 : Constant  Value=-g*Vehicle.Airframe.mass  OutDataTypeStr=single  SampleTime=Ts
  altitude_cmd : Outport  VectorParamsAs1DForOutWhenUnconnected=off
  wires:
  Sum3/1 -> P_z/1  "errZ"
  TakeoffOrControl_Switch/1 -> Sum4/2
  Bus Selector6/1 -> Sum3/2  "<Z>"
  Bus Selector6/2 -> D_z/1  "<dz>"
  w0/1 -> Sum4/1, takeoff_gain/1
  D_z/1 -> Sum15/2  "dz"
  takeoff_gain/1 -> TakeoffOrControl_Switch/1
  takeoff_flag/1 -> TakeoffOrControl_Switch/2
  PosZ/1 -> Sum3/1
  P_z/1 -> Sum15/1
  Sum15/1 -> TakeoffOrControl_Switch/3
  Sum4/1 -> SaturationThrust/1
  SaturationThrust/1 -> altitude_cmd/1
  states_estim/1 -> Bus Selector6/1

== system flightController/Flight Controller/thrustsToMotorCommands ==
  thrusts_refin : Inport
  MotorDirections : Gain  Gain=[1 -1 1 -1]
  Saturation5 : Saturate  UpperLimit=Vehicle.Motor.maxLimit  LowerLimit=Vehicle.Motor.minLimit
  ThrustToMotorCommand : Gain  Gain=-Vehicle.Motor.thrustToMotorCommand
  motors_cmdout : Outport  VectorParamsAs1DForOutWhenUnconnected=off
  wires:
  Saturation5/1 -> MotorDirections/1
  MotorDirections/1 -> motors_cmdout/1
  ThrustToMotorCommand/1 -> Saturation5/1
  thrusts_refin/1 -> ThrustToMotorCommand/1

== system flightController/Variant Subsystem/ANN ==
  note: PREPROCESAMIENTO
  note: Normalizacion
  ReferenceValueServerBus : Inport
  states_estim : Inport  Port=2
  Sensores : Inport  Port=3
  Delay1 : Delay  Commented=on  DelayLength=1  InitialCondition=0
  Delay2 : Delay  Commented=on  DelayLength=1  InitialCondition=0
  Delay3 : Delay  Commented=on  DelayLength=1  InitialCondition=0
  Mux : Mux  Commented=on
  Predict : deeplib/Predict  Commented=on  Network=Network from MAT-file  NetworkFunction=squeezenet  NetworkFilePath=C:\Users\Eduardo\Documents\universidad\Tesis\Modelos\net.mat  MiniBatchSize=50  InputDataFormats={ '', '' }  Predictions=on  Activations={}  ForceInterpretedSim=off  EnableDLNetwork=off
      settings: SourceProductBaseCode=NN
  Predict1 : deeplib/Predict  Network=Network from MAT-file  NetworkFunction=squeezenet  NetworkFilePath=C:\Users\Eduardo\Documents\universidad\Tesis\Modelos\net.mat  MiniBatchSize=50  InputDataFormats={ '', '' }  Predictions=on  Activations={}  ForceInterpretedSim=off  EnableDLNetwork=off
      settings: SourceProductBaseCode=NN
  Reshape : Reshape  Commented=on  OutputDimensionality=Customize  OutputDimensions=[1,72]
  Reshape1 : Reshape  OutputDimensionality=Customize  OutputDimensions=[1,72]
  Scope{1..5} (5 alike) : Scope  Commented=on
  Subsystem : Subsystem  Commented=on
  Subsystem2 : Subsystem
  Subsystem3 : Subsystem
  Subsystem4 : Subsystem  Commented=on
  To Workspace : ToWorkspace  Commented=on  VariableName=Input1  SampleTime=-1
      settings: Save2DSignal=2-D array (concatenate along first dimension)
  To Workspace1 : ToWorkspace  Commented=on  VariableName=Out_Net1  SampleTime=-1
      settings: Save2DSignal=2-D array (concatenate along first dimension)
  To Workspace2 : ToWorkspace  VariableName=Out_Net  SampleTime=-1
      settings: Save2DSignal=2-D array (concatenate along first dimension)
  To Workspace3 : ToWorkspace  VariableName=Input  SampleTime=-1
      settings: Save2DSignal=2-D array (concatenate along first dimension)
  motors_refout : Outport
  wires:
  Subsystem2/1(Output) -> Reshape1/1
  Predict1/1 -> Subsystem3/1(In1), To Workspace2/1
  Sensores/1 -> Subsystem2/3(In3)
  states_estim/1 -> Subsystem2/2(In2)
  Reshape1/1 -> Predict1/1, To Workspace3/1
  ReferenceValueServerBus/1 -> Subsystem2/1(In1)
  Subsystem3/1(motors_refout) -> motors_refout/1
  Predict/1 -> To Workspace1/1, Subsystem4/1(In1)
  Reshape/1 -> To Workspace/1, Predict/1
  Subsystem4/1(motors_refout) -> Scope5/1
  Subsystem/1(Norm_States) -> Scope1/1, Mux/1, Delay1/1
  Mux/1 -> Reshape/1
  Delay1/1 -> Mux/2, Scope2/1, Delay2/1
  Delay2/1 -> Mux/3, Scope3/1, Delay3/1
  Delay3/1 -> Scope4/1, Mux/4

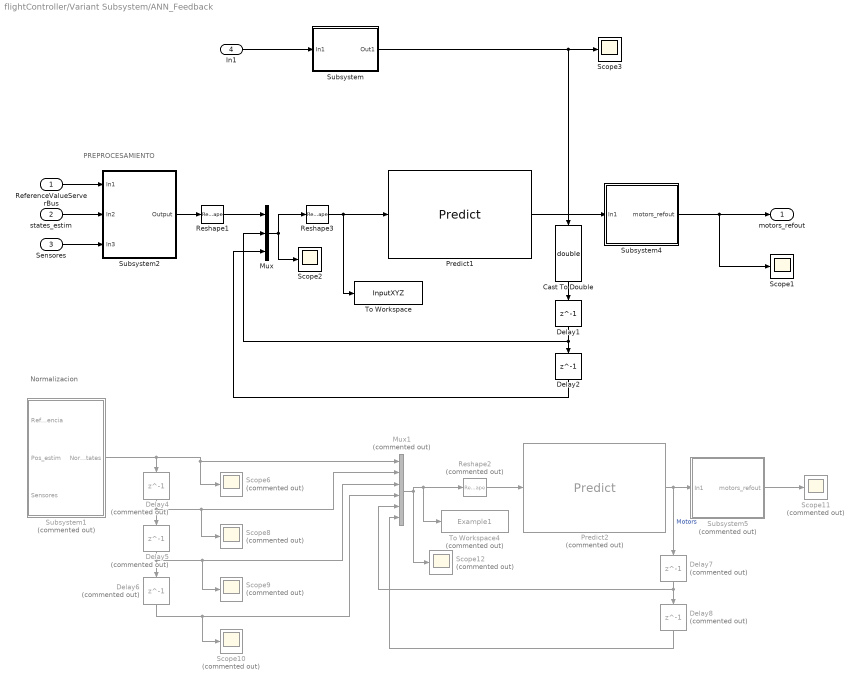
== system flightController/Variant Subsystem/ANN_Feedback ==
  note: Normalizacion
  note: PREPROCESAMIENTO
  ReferenceValueServerBus : Inport
  states_estim : Inport  Port=2
  Sensores : Inport  Port=3
  In1 : Inport  Port=4
  Cast To Double : DataTypeConversion  OutDataTypeStr=double
  Delay1 : Delay  DelayLength=1  InitialCondition=0
  Delay2 : Delay  DelayLength=1  InitialCondition=0
  Delay{4..8} (5 alike) : Delay  Commented=on  DelayLength=1  InitialCondition=0
  Mux : Mux  Inputs=3
  Mux1 : Mux  Commented=on  Inputs=6
  Predict1 : deeplib/Predict  Network=Network from MAT-file  NetworkFunction=squeezenet  NetworkFilePath=C:\Users\Eduardo\MATLAB\Projects\examples\Training\Models\net.mat  MiniBatchSize=50  InputDataFormats={ '', '' }  Predictions=on  Activations={}  ForceInterpretedSim=off  EnableDLNetwork=off
      settings: SourceProductBaseCode=NN
  Predict2 : deeplib/Predict  Commented=on  Network=Network from MAT-file  NetworkFunction=squeezenet  NetworkFilePath=C:\Users\Eduardo\Documents\universidad\Tesis\Modelos\net.mat  MiniBatchSize=50  InputDataFormats={ '', '' }  Predictions=on  Activations={}  ForceInterpretedSim=off  EnableDLNetwork=off
      settings: SourceProductBaseCode=NN
  Reshape1 : Reshape  OutputDimensionality=Customize  OutputDimensions=[1,length(sts_cnames)*(delays+1)]
  Reshape2 : Reshape  Commented=on  OutputDimensionality=Customize  OutputDimensions=[1,88]
  Reshape3 : Reshape  OutputDimensionality=Customize  OutputDimensions=[1,(length(sts_cnames)*(delays+1))+8]
  Scope1 : Scope
  Scope{6,8..12} (6 alike) : Scope  Commented=on
  Scope2 : Scope
  Scope3 : Scope
  Subsystem : Subsystem
  Subsystem1 : Subsystem  Commented=on
  Subsystem2 : Subsystem
  Subsystem4 : Subsystem
  Subsystem5 : Subsystem  Commented=on
  To Workspace : ToWorkspace  VariableName=InputXYZ  SampleTime=-1
      settings: Save2DSignal=2-D array (concatenate along first dimension)
  To Workspace4 : ToWorkspace  Commented=on  VariableName=Example1  SaveFormat=Structure With Time  SampleTime=-1
  motors_refout : Outport
  wires:
  Delay8/1 -> Mux1/6
  Delay7/1 -> Mux1/5, Delay8/1
  Subsystem1/1(Norm_States) -> Scope6/1, Mux1/1, Delay4/1
  Mux1/1 -> Reshape2/1, To Workspace4/1, Scope12/1
  Delay5/1 -> Mux1/3, Scope9/1, Delay6/1
  Delay6/1 -> Scope10/1, Mux1/4
  Reshape2/1 -> Predict2/1
  Delay4/1 -> Mux1/2, Scope8/1, Delay5/1
  Predict2/1 -> Delay7/1, Subsystem5/1(In1)  "Motors"
  Subsystem5/1(motors_refout) -> Scope11/1
  states_estim/1 -> Subsystem2/2(In2)
  Sensores/1 -> Subsystem2/3(In3)
  Reshape1/1 -> Mux/1
  ReferenceValueServerBus/1 -> Subsystem2/1(In1)
  Subsystem2/1(Output) -> Reshape1/1
  Delay1/1 -> Mux/2, Delay2/1
  Mux/1 -> Reshape3/1, Scope2/1
  Delay2/1 -> Mux/3
  Reshape3/1 -> Predict1/1, To Workspace/1
  In1/1 -> Subsystem/1(In1)
  Subsystem/1(Out1) -> Cast To Double/1, Scope3/1
  Predict1/1 -> Subsystem4/1(In1)
  Subsystem4/1(motors_refout) -> Scope1/1, motors_refout/1
  Cast To Double/1 -> Delay1/1

== system flightController/Variant Subsystem/LSTM ==
  note: PREPROCESAMIENTO
  note: PREPROCESAMIENTO
  ReferenceValueServerBus : Inport
  states_estim : Inport  Port=2
  Sensores : Inport  Port=3
  Delay : Delay  Commented=on  DelayLength=1
  Delay1 : Delay  Commented=on
  Delay2 : Delay  Commented=on  DelayLength=3
  Mux1 : Mux  Commented=on  Inputs=3
  Predict : deeplib/Predict  Network=Network from MATLAB function  NetworkFunction=myprediction  NetworkFilePath=mypre  MiniBatchSize=1024  InputDataFormats={ '', '' }  Predictions=on  Activations={}  ForceInterpretedSim=off  EnableDLNetwork=on
      settings: SourceProductBaseCode=NN
  ReferenceValueServerBus1 : InportShadow
  Scope8 : Scope
  Sensores1 : InportShadow  Port=3
  Subsystem1 : Subsystem
  Subsystem2 : Subsystem
  Subsystem3 : Subsystem  Commented=on
  Terminator : Terminator  Commented=on
  To Workspace : ToWorkspace  VariableName=Test  SaveFormat=Structure With Time  SampleTime=5e-3
  states_estim1 : InportShadow  Port=2
  motors_refout : Outport
  wires:
  Subsystem3/1(Output) -> Terminator/1
  Subsystem2/1(Output) -> To Workspace/1, Predict/1
  ReferenceValueServerBus/1 -> Subsystem2/1(In1)
  Delay1/1 -> Mux1/2
  Subsystem1/1(motors_refout) -> motors_refout/1, Scope8/1
  Sensores/1 -> Subsystem2/3(In3)
  states_estim1/1 -> Subsystem3/2(In2)
  ReferenceValueServerBus1/1 -> Subsystem3/1(In1)
  states_estim/1 -> Subsystem2/2(In2)
  Delay2/1 -> Mux1/3
  Delay/1 -> Mux1/1
  Sensores1/1 -> Subsystem3/3(In3)
  Predict/1 -> Delay/1, Delay2/1, Delay1/1, Subsystem1/1(In1)
  Mux1/1 -> Subsystem3/4(In4)

== system flightController/Flight Controller/MOTOR 1 /PITCH  ==
  Step6 : Step  Time=0.001  Before=30  After=350
  Step7 : Step  Time=0.001  Before=30  After=380
  Step8 : Step  Time=1.5  Before=1  After=0
  Switch2 : Switch  Criteria=u2 > Threshold
  Out1 : Outport
  wires:
  Switch2/1 -> Out1/1
  Step8/1 -> Switch2/2
  Step7/1 -> Switch2/3
  Step6/1 -> Switch2/1

== system flightController/Flight Controller/MOTOR 1 /ROLL  ==
  Step10 : Step  Time=0.001  Before=30  After=380
  Step11 : Step  Time=1.5  Before=1  After=0
  Step9 : Step  Time=0.001  Before=30  After=350
  Switch3 : Switch  Criteria=u2 > Threshold
  Out1 : Outport
  wires:
  Step9/1 -> Switch3/1
  Step10/1 -> Switch3/3
  Step11/1 -> Switch3/2
  Switch3/1 -> Out1/1

== system flightController/Flight Controller/MOTOR 1 /SUBIR ==
  note: SI
  Pulse Generator1 : DiscretePulseGenerator  PulseType=Time based  Amplitude=30  Period=1.5  PulseWidth=50
  Step1 : Step  Time=0.001  Before=30  After=350
  Step3 : Step  Time=1.5  Before=1  After=0
  Step4 : Step  Time=0.001  Before=-30  After=237
  Sum1 : Sum  Inputs=|+-
  Switch1 : Switch  Criteria=u2 > Threshold
  Out1 : Outport
  wires:
  Pulse Generator1/1 -> Sum1/2
  Sum1/1 -> Switch1/3
  Step3/1 -> Switch1/2
  Step4/1 -> Sum1/1
  Step1/1 -> Switch1/1
  Switch1/1 -> Out1/1

== system flightController/Flight Controller/MOTOR 1 /YAW ==
  Pulse Generator : DiscretePulseGenerator  PulseType=Time based  Amplitude=50  Period=1.5  PulseWidth=50
  Step : Step  Time=0.001  Before=30  After=350
  Step2 : Step  Time=0.001  Before=30  After=420
  Step5 : Step  Time=1.5  Before=1  After=0
  Sum : Sum  Inputs=|+-
  Switch : Switch  Criteria=u2 > Threshold
  Out1 : Outport
  wires:
  Step/1 -> Switch/1
  Step5/1 -> Switch/2
  Sum/1 -> Switch/3
  Step2/1 -> Sum/1
  Pulse Generator/1 -> Sum/2
  Switch/1 -> Out1/1

== system flightController/Flight Controller/MOTOR 2/PITCH  ==
  Step6 : Step  Time=0.001  Before=-30  After=-380
  Step8 : Step  Time=0.001  Before=-30  After=-350
  Step9 : Step  Time=1.5
  Switch2 : Switch  Criteria=u2 > Threshold
  Out1 : Outport
  wires:
  Switch2/1 -> Out1/1
  Step9/1 -> Switch2/2
  Step8/1 -> Switch2/3
  Step6/1 -> Switch2/1

== system flightController/Flight Controller/MOTOR 2/ROLL ==
  Step10 : Step  Time=0.001  Before=-30  After=-310
  Step11 : Step  Time=0.001  Before=-30  After=-350
  Step12 : Step  Time=1.5
  Switch3 : Switch  Criteria=u2 > Threshold
  Out1 : Outport
  wires:
  Switch3/1 -> Out1/1
  Step10/1 -> Switch3/1
  Step11/1 -> Switch3/3
  Step12/1 -> Switch3/2

== system flightController/Flight Controller/MOTOR 2/SUBIR ==
  note: SI
  Pulse Generator1 : DiscretePulseGenerator  PulseType=Time based  Amplitude=30  Period=1.5  PulseWidth=50
  Step4 : Step  Time=0.001  Before=-30  After=-350
  Step5 : Step  Time=1.5
  Step7 : Step  Time=0.001  Before=-30  After=-237
  Sum1 : Sum  Inputs=|++
  Switch : Switch  Criteria=u2 > Threshold
  Out1 : Outport
  wires:
  Switch/1 -> Out1/1
  Pulse Generator1/1 -> Sum1/2
  Step4/1 -> Switch/3
  Step7/1 -> Sum1/1
  Step5/1 -> Switch/2
  Sum1/1 -> Switch/1

== system flightController/Flight Controller/MOTOR 2/YAW ==
  Pulse Generator : DiscretePulseGenerator  PulseType=Time based  Amplitude=50  Period=1.5  PulseWidth=50
  Step1 : Step  Time=0.001  Before=-30  After=-280
  Step2 : Step  Time=0.001  Before=-30  After=-350
  Step3 : Step  Time=1.5
  Sum : Sum  Inputs=|++
  Switch1 : Switch  Criteria=u2 > Threshold
  Out1 : Outport
  wires:
  Switch1/1 -> Out1/1
  Step2/1 -> Switch1/3
  Step1/1 -> Sum/2
  Sum/1 -> Switch1/1
  Pulse Generator/1 -> Sum/1
  Step3/1 -> Switch1/2

== system flightController/Flight Controller/MOTOR 3 /PITCH  ==
  Step6 : Step  Time=0.001  Before=30  After=350
  Step7 : Step  Time=0.001  Before=30  After=310
  Step8 : Step  Time=1.5  Before=1  After=0
  Switch2 : Switch  Criteria=u2 > Threshold
  Out1 : Outport
  wires:
  Switch2/1 -> Out1/1
  Step6/1 -> Switch2/1
  Step8/1 -> Switch2/2
  Step7/1 -> Switch2/3

== system flightController/Flight Controller/MOTOR 3 /ROLL  ==
  Step10 : Step  Time=0.001  Before=30  After=310
  Step11 : Step  Time=1.5  Before=1  After=0
  Step9 : Step  Time=0.001  Before=30  After=350
  Switch3 : Switch  Criteria=u2 > Threshold
  Out1 : Outport
  wires:
  Switch3/1 -> Out1/1
  Step10/1 -> Switch3/3
  Step11/1 -> Switch3/2
  Step9/1 -> Switch3/1

== system flightController/Flight Controller/MOTOR 3 /SUBIR ==
  note: SI
  Pulse Generator1 : DiscretePulseGenerator  PulseType=Time based  Amplitude=30  Period=1.5  PulseWidth=50
  Step : Step  Time=0.001  Before=30  After=350
  Step4 : Step  Time=0.001  Before=-30  After=237
  Step5 : Step  Time=1.5  Before=1  After=0
  Sum1 : Sum  Inputs=|+-
  Switch : Switch  Criteria=u2 > Threshold
  Out1 : Outport
  wires:
  Switch/1 -> Out1/1
  Pulse Generator1/1 -> Sum1/2
  Sum1/1 -> Switch/3
  Step4/1 -> Sum1/1
  Step/1 -> Switch/1
  Step5/1 -> Switch/2

== system flightController/Flight Controller/MOTOR 3 /YAW ==
  Pulse Generator : DiscretePulseGenerator  PulseType=Time based  Amplitude=50  Period=1.5  PulseWidth=50
  Step1 : Step  Time=0.001  Before=30  After=350
  Step2 : Step  Time=0.001  Before=30  After=420
  Step3 : Step  Time=1.5  Before=1  After=0
  Sum : Sum  Inputs=|+-
  Switch1 : Switch  Criteria=u2 > Threshold
  Out1 : Outport
  wires:
  Switch1/1 -> Out1/1
  Step3/1 -> Switch1/2
  Step1/1 -> Switch1/1
  Pulse Generator/1 -> Sum/2
  Sum/1 -> Switch1/3
  Step2/1 -> Sum/1

== system flightController/Flight Controller/MOTOR 4 /PITCH  ==
  Step6 : Step  Time=0.001  Before=-30  After=-310
  Step8 : Step  Time=0.001  Before=-30  After=-350
  Step9 : Step  Time=1.5
  Switch2 : Switch  Criteria=u2 > Threshold
  Out1 : Outport
  wires:
  Switch2/1 -> Out1/1
  Step9/1 -> Switch2/2
  Step8/1 -> Switch2/3
  Step6/1 -> Switch2/1

== system flightController/Flight Controller/MOTOR 4 /ROLL  ==
  Step10 : Step  Time=0.001  Before=-30  After=-380
  Step11 : Step  Time=0.001  Before=-30  After=-350
  Step12 : Step  Time=1.5
  Switch3 : Switch  Criteria=u2 > Threshold
  Out1 : Outport
  wires:
  Switch3/1 -> Out1/1
  Step11/1 -> Switch3/3
  Step10/1 -> Switch3/1
  Step12/1 -> Switch3/2

== system flightController/Flight Controller/MOTOR 4 /SUBIR ==
  note: SI
  Pulse Generator1 : DiscretePulseGenerator  PulseType=Time based  Amplitude=30  Period=1.5  PulseWidth=50
  Step4 : Step  Time=0.001  Before=-30  After=-350
  Step5 : Step  Time=1.5
  Step7 : Step  Time=0.001  Before=-30  After=-237
  Sum1 : Sum  Inputs=|++
  Switch : Switch  Criteria=u2 > Threshold
  Out1 : Outport
  wires:
  Switch/1 -> Out1/1
  Sum1/1 -> Switch/1
  Step7/1 -> Sum1/1
  Step4/1 -> Switch/3
  Pulse Generator1/1 -> Sum1/2
  Step5/1 -> Switch/2

== system flightController/Flight Controller/MOTOR 4 /YAW ==
  Pulse Generator : DiscretePulseGenerator  PulseType=Time based  Amplitude=50  Period=1.5  PulseWidth=50
  Step1 : Step  Time=0.001  Before=-30  After=-280
  Step2 : Step  Time=0.001  Before=-30  After=-350
  Step3 : Step  Time=1.5
  Sum : Sum  Inputs=|++
  Switch1 : Switch  Criteria=u2 > Threshold
  Out1 : Outport
  wires:
  Switch1/1 -> Out1/1
  Sum/1 -> Switch1/1
  Pulse Generator/1 -> Sum/1
  Step2/1 -> Switch1/3
  Step1/1 -> Sum/2
  Step3/1 -> Switch1/2
